simulink model "Platform_way_points_planner"  (R2025b)
settings: Solver=VariableStepAuto  StartTime=0.0  StopTime=100  FixedStep=0.1  MaxStep=1/2000  RelTol=1e-3
libraries: MISSILE_GUIDANCE_LIB2 x3, simulink_extras x1
settings Model: PacingRate=11  Creator=Leonid  LastModifiedBy=Leonid

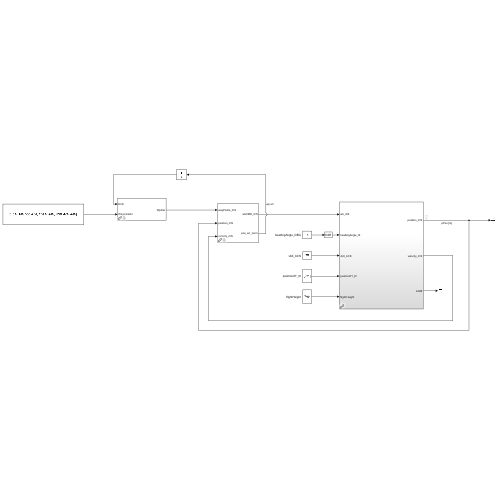
[thumbnail: Simulink's stored preview of the top-level diagram]
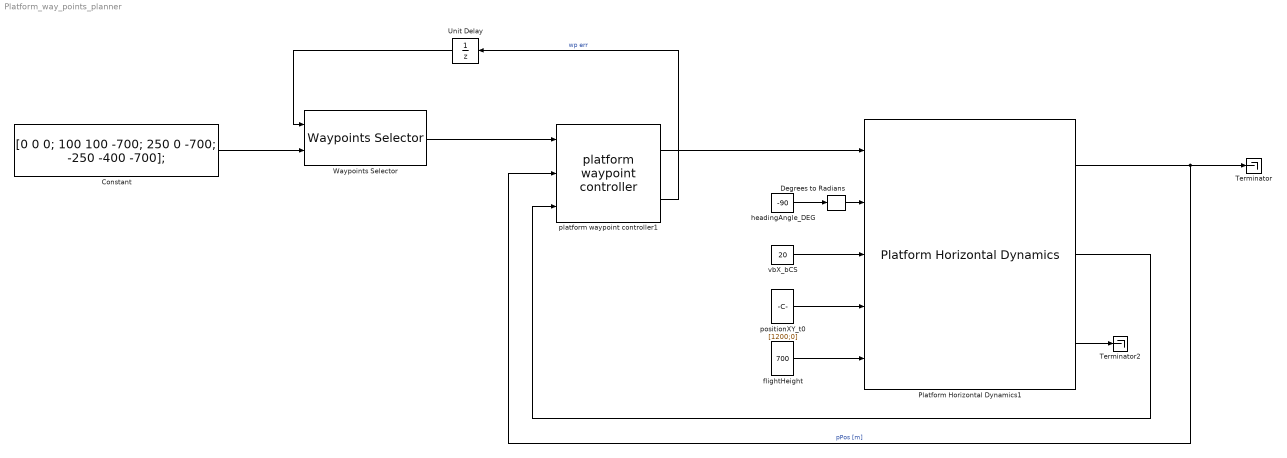
== system Platform_way_points_planner ==
  Constant : Constant  Value=[0 0 0; 100 100 -700; 250 0 -700; -250 -400 -700];
  Degrees to Radians : simulink_extras/Transformations/Degrees to Radians
  Platform Horizontal Dynamics1 : MISSILE_GUIDANCE_LIB2/Platform Horizontal Dynamics  SystemSampleTime=-1  VariantActivationTime=update diagram  EmptyChoice=off  PassThrough=off  PassThroughVariantControl=(default)  EmptyChoiceVariantControl=(default)  AllowFlexibleInterface=on  Latency=0  AutoFrameSizeCalculation=off
  Terminator : Terminator
  Terminator2 : Terminator
  Unit Delay : UnitDelay  SampleTime=-1  HasFrameUpgradeWarning=on
  Waypoints Selector : MISSILE_GUIDANCE_LIB2/Waypoints Selector  threshold=2
  flightHeight : Constant  Value=700  VectorParams1D=off
  headingAngle_DEG : Constant  Value=-90  VectorParams1D=off
  platform waypoint controller1 : MISSILE_GUIDANCE_LIB2/platform waypoint controller  K=1
  positionXY_t0 : Constant  Value=[1200;0]  VectorParams1D=off
  vbX_bCS : Constant  Value=20
  wires:
  Degrees to Radians/1 -> Platform Horizontal Dynamics1/2
  Platform Horizontal Dynamics1/1 -> platform waypoint controller1/2, Terminator/1  "pPos [m]"
  headingAngle_DEG/1 -> Degrees to Radians/1
  vbX_bCS/1 -> Platform Horizontal Dynamics1/3
  positionXY_t0/1 -> Platform Horizontal Dynamics1/4
  flightHeight/1 -> Platform Horizontal Dynamics1/5
  Platform Horizontal Dynamics1/2 -> platform waypoint controller1/3
  Platform Horizontal Dynamics1/3 -> Terminator2/1
  platform waypoint controller1/2 -> Unit Delay/1  "wp err"
  Waypoints Selector/1 -> platform waypoint controller1/1
  platform waypoint controller1/1 -> Platform Horizontal Dynamics1/1
  Constant/1 -> Waypoints Selector/2
  Unit Delay/1 -> Waypoints Selector/1
